simulink model "Msimlab3_1"  (R2021a)
settings: Solver=VariableStepAuto  StartTime=0.0  StopTime=18  MaxStep=1e-4  RelTol=1e-3
values from neighbouring files (symbols this model uses):
  a = 0:0.5:1    [p1.m]
undefined symbols (not defined in the file or in its folder): i
libraries: simulink x1
settings Model: Creator=danie  LastModifiedBy=ruipe
settings SolverCC: ZeroCrossAlgorithm=Adaptive  AlgebraicLoopSolver=TrustRegion
settings DebuggingCC: IgnoredZcDiagnostic=none  SFMachineParentedDataDiag=warning

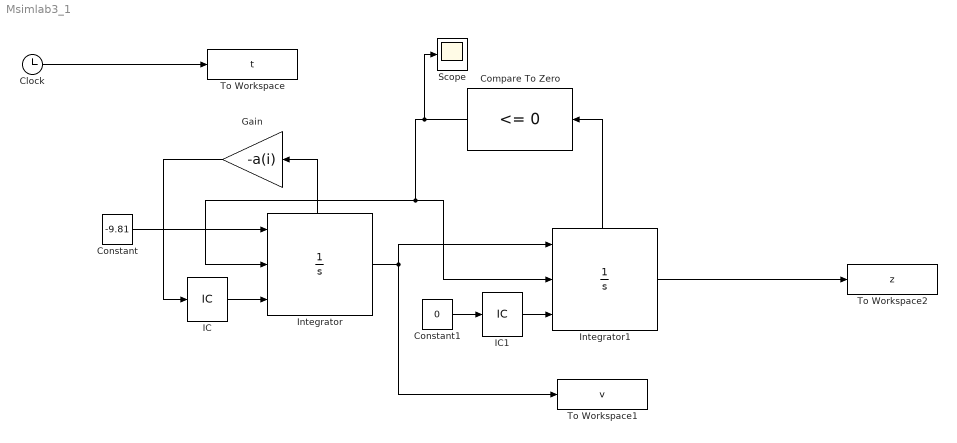
== system Msimlab3_1 ==
  Clock : Clock
  Compare To Zero : simulink/Logic and Bit Operations/Compare To Zero  relop=<=  OutDataTypeStr=boolean
  Constant : Constant  Description=Gravidade  Value=-9.81
      settings: AttributesFormatString=Gravidade
  Constant1 : Constant  Description=Pavimento  Value=0
      settings: AttributesFormatString=Pavimento
  Gain : Gain  Description=Elasticidade da bola  Gain=-a(i)
      settings: AttributesFormatString=Elasticidade da bola
  IC : InitialCondition  Description=Velocidade inicial  Value=0
      settings: AttributesFormatString=Velocidade inicial
  IC1 : InitialCondition  Description=Posição inicial  Value=10
      settings: AttributesFormatString=Posição inicial
  Integrator : Integrator  ExternalReset=level hold  InitialConditionSource=external  ShowStatePort=on
      settings: AttributesFormatString=Velocidade
  Integrator1 : Integrator  ExternalReset=rising  InitialConditionSource=external  LimitOutput=on  ShowStatePort=on
      settings: AttributesFormatString=Posição
  Scope : Scope
  To Workspace : ToWorkspace  VariableName=t  SaveFormat=Timeseries  SampleTime=-1
      settings: Save2DSignal=2-D array (concatenate along first dimension)
  To Workspace1 : ToWorkspace  VariableName=v  SaveFormat=Timeseries  SampleTime=-1
      settings: Save2DSignal=2-D array (concatenate along first dimension)
  To Workspace2 : ToWorkspace  VariableName=z  SaveFormat=Timeseries  SampleTime=-1
      settings: Save2DSignal=2-D array (concatenate along first dimension)
  wires:
  IC/1 -> Integrator/3
  IC1/1 -> Integrator1/3
  Constant1/1 -> IC1/1
  Integrator/State -> Gain/1
  Gain/1 -> IC/1
  Integrator/1 -> To Workspace1/1, Integrator1/1
  Integrator1/State -> Compare To Zero/1
  Compare To Zero/1 -> Scope/1, Integrator1/2, Integrator/2
  Constant/1 -> Integrator/1
  Clock/1 -> To Workspace/1
  Integrator1/1 -> To Workspace2/1
